simulink model "AdaptivePID"  (R2018a)
settings: Solver=VariableStepAuto  StartTime=0.0  StopTime=10.0  RelTol=1e-3
undefined symbols (not defined in the file): a, Gamma, Ps
settings Model: Creator=Gupta  LastModifiedBy=Gupta

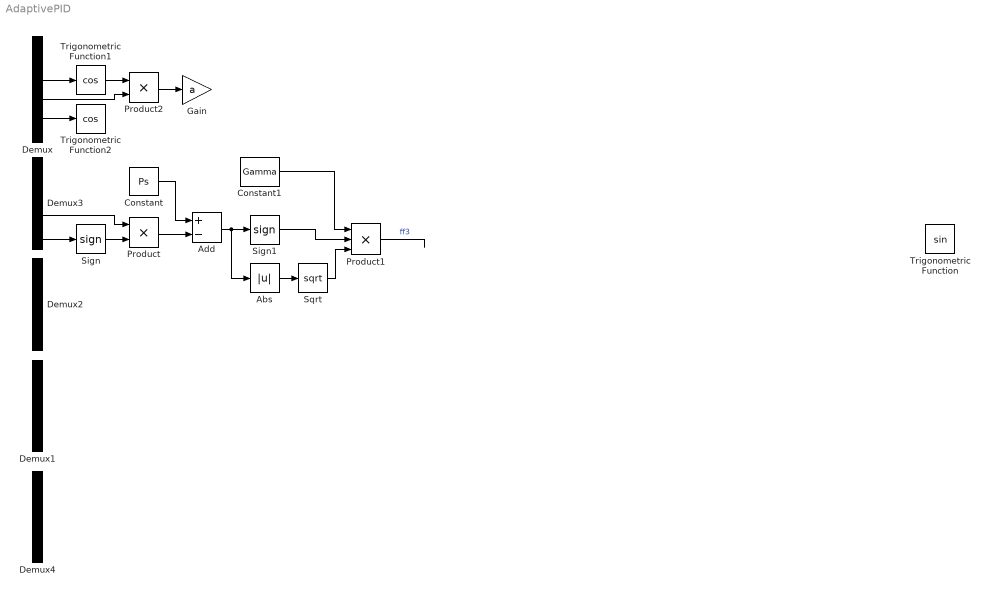
== system AdaptivePID ==
  Abs : Abs
  Add : Sum  Inputs=+-
  Constant : Constant  Value=Ps
  Constant1 : Constant  Value=Gamma
  Demux : Demux  Outputs=6
  Demux{1..4} (4 alike) : Demux
  Gain : Gain  Gain=a
  Product : Product
  Product1 : Product  Inputs=3
  Product2 : Product
  Sign : Signum
  Sign1 : Signum
  Sqrt : Sqrt  SaturateOnIntegerOverflow=on
  Trigonometric Function : Trigonometry
  Trigonometric Function1 : Trigonometry  Operator=cos
  Trigonometric Function2 : Trigonometry  Operator=cos
  wires:
  Demux3/4 -> Sign/1
  Sign/1 -> Product/2
  Demux3/3 -> Product/1
  Product/1 -> Add/2
  Constant/1 -> Add/1
  Add/1 -> Abs/1, Sign1/1
  Abs/1 -> Sqrt/1
  Sqrt/1 -> Product1/3
  Sign1/1 -> Product1/2
  Constant1/1 -> Product1/1
  Product1/1 -> ?  "ff3"
  Demux/3 -> Trigonometric Function1/1
  Trigonometric Function1/1 -> Product2/1
  Demux/4 -> Product2/2
  Product2/1 -> Gain/1
  Demux/5 -> Trigonometric Function2/1
